simulink model "Suspension_system"  (R2023a)
settings: Solver=VariableStepAuto  StartTime=0.0  StopTime=10.0  RelTol=1e-3
values from neighbouring files (symbols this model uses):
  amp = 0.0025    [Parameters.m]
  c = 650    [Parameters.m]
  D_amp = 0.015    [Parameters.m]
  D_flat = 1    [Parameters.m]
  D_wave = 0.05    [Parameters.m]
  T_flat = 0.3048    [Parameters.m]    (also in task3.m; task4.m = 1)
  T_wave = 0.01    [Parameters.m]    (also in task3.m; task4.m = 0.05)
libraries: fl_lib x7, nesl_utility x4, simulink x1
settings Model: Creator=arnin  LastModifiedBy=arnin

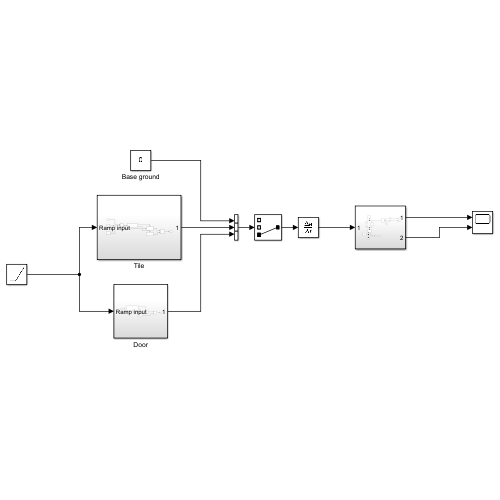
[thumbnail: Simulink's stored preview of the top-level diagram]
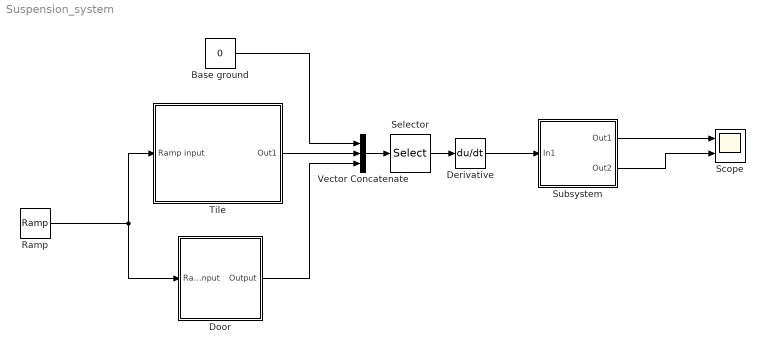
== system Suspension_system ==
  Base ground : Constant  Value=0
  Derivative : Derivative
  Door : Subsystem
  Ramp : simulink/Sources/Ramp  slope=3  start=0  InitialOutput=0
  Scope : Scope  NumInputPorts=2
  Selector : Selector  InputPortWidth=3  IndexOptions=Index vector (dialog)  Indices=[3]  OutputSizes=1
  Subsystem : Subsystem
  Tile : Subsystem
  Vector Concatenate : Concatenate  NumInputs=3
  wires:
  Ramp/1 -> Door/1(Ramp input), Tile/1(Ramp input)
  Base ground/1 -> Vector Concatenate/1
  Tile/1(Out1) -> Vector Concatenate/2
  Door/1(Output) -> Vector Concatenate/3
  Vector Concatenate/1 -> Selector/1
  Derivative/1 -> Subsystem/1(In1)
  Selector/1 -> Derivative/1
  Subsystem/1(Out1) -> Scope/1
  Subsystem/2(Out2) -> Scope/2

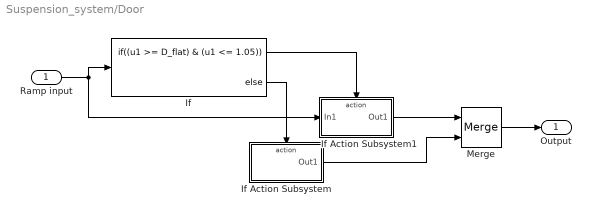
== system Suspension_system/Door ==
  Ramp input : Inport
  If : If  IfExpression=(u1 >= D_flat) & (u1 <= 1.05)
  If Action Subsystem : Subsystem  TreatAsAtomicUnit=on
  If Action Subsystem1 : Subsystem  TreatAsAtomicUnit=on
  Merge : Merge
  Output : Outport
  wires:
  If/2 -> If Action Subsystem/Action
  If Action Subsystem1/1(Out1) -> Merge/1
  Ramp input/1 -> If Action Subsystem1/1(In1), If/1
  If Action Subsystem/1(Out1) -> Merge/2
  If/1 -> If Action Subsystem1/Action
  Merge/1 -> Output/1

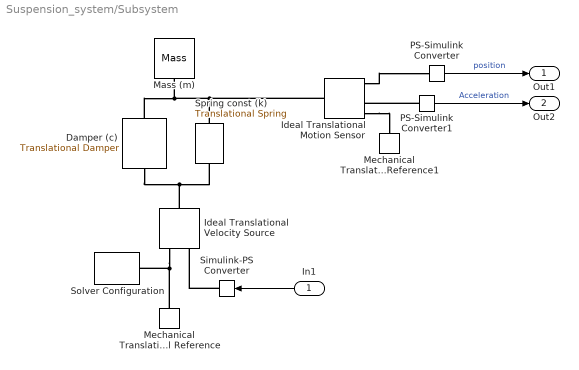
== system Suspension_system/Subsystem ==
  In1 : Inport
  Damper (c) : fl_lib/Mechanical/Translational Elements/Translational Damper  D=c N*s/m  v_specify=off  v_priority=None  v=0 m/s  v_nominal_specify=off  v_nominal_unit=m/s  v_nominal_value=1  f_specify=off  f_priority=None  f=0 N  f_nominal_specify=off  f_nominal_unit=N  f_nominal_value=1
  Ideal Translational Motion Sensor : fl_lib/Mechanical/Mechanical Sensors/Ideal Translational Motion Sensor  reference=foundation.enum.MeasurementReference.difference  acceleration_port=true  velocity_port=true  position_port=true  offset=0 m
      settings: InternalSimscapePortConfiguration="{\"Bottom\":[],\"Left\":[{\"id\":\"R\",\"label\":\"R\",\"type\":\"foundation.mechanical.translational.translational\"}],\"Right\":[{\"id\":\"C\",\"label\":\"C\",\"type\":\"foundation.mechanical.translational.translational\"},{\"id\":\"A\",\"label\":\"A\",\"type\":\"output\"},{\"id\":\"V\",\"label\":\"V\",\"type\":\"output\"},{\"id\":\"P\",\"label\":\"P\",\"type\":\"output\"}],\"Top\":[]}"
  Ideal Translational Velocity Source : fl_lib/Mechanical/Mechanical Sources/Ideal Translational Velocity Source
  Mass (m) : fl_lib/Mechanical/Translational Elements/Mass  mass=M kg  num_ports=foundation.enum.numPorts2.one  v_specify=off  v_priority=High  v=0 m/s  v_nominal_specify=off  v_nominal_unit=m/s  v_nominal_value=1  f_specify=off  f_priority=None  f=0 N  f_nominal_specify=off  f_nominal_unit=N  f_nominal_value=1
  Mechanical Translational Reference : fl_lib/Mechanical/Translational Elements/Mechanical Translational Reference
  Mechanical Translational Reference1 : fl_lib/Mechanical/Translational Elements/Mechanical Translational Reference
  PS-Simulink Converter : nesl_utility/PS-Simulink Converter  PhysicalDomain=network_engine_domain  SubClassName=ps_output  LeftPortType=input  RightPortType=output  PseudoPeriodic=off  Frequencies=[]  VectorFormat=inherit  Unit=inherit  AffineConversion=off
  PS-Simulink Converter1 : nesl_utility/PS-Simulink Converter  PhysicalDomain=network_engine_domain  SubClassName=ps_output  LeftPortType=input  RightPortType=output  PseudoPeriodic=off  Frequencies=[]  VectorFormat=inherit  Unit=inherit  AffineConversion=off
  Simulink-PS Converter : nesl_utility/Simulink-PS Converter  PhysicalDomain=network_engine_domain  SubClassName=ps_input  LeftPortType=input  RightPortType=output  PseudoPeriodic=off  Frequencies=[]  NoiseDistribution=none  NoiseParameters=[]  Unit=1  AffineConversion=off  FilteringAndDerivatives=provide  SimscapeFilterOrder=1  InputFilterTimeConstant=0.001  UdotUserProvided=0
  Solver Configuration : nesl_utility/Solver Configuration  PhysicalDomain=network_engine_domain  SubClassName=solver  LeftPortType=input  RightPortType=generic  Tones=[]  Harmonics=[]  SimulateNoise=off  Profile=off  UseLocalSampling=off  EnableSwitchedLinearOptims=on  FrequencyDomain=off  UseCCode=off  RelTol=0.001  AbsTol=0.001  MinStep=1e-09  ToWorkspace=off  RevertToSquareIcSolve=off  NumHomotopyIterations=100  PhasorMode=off  PhasorModeNumHarmonics=1  ConsistencySolver=NEWTON_XTOL_AFTER_FTOL  IndexReductionMethod=DerivativeReplacement  DoDC=off  ResidualTolerance=1e-09  ConsistencyTolSource=GLOBAL  ConsistencyAbsTol=0.001  ConsistencyRelTol=0.001  ConsistencyTolFactor=0.001  UseLocalSolver=off  LocalSolverChoice=NE_BACKWARD_EULER_ADVANCER  ResolveIndetEquations=on  FunctionEvalNumThread=1  LocalSolverSampleTime=0.001  DoFixedCost=off  MaxNonlinIter=3  MaxModeIter=2  ComputeImpulses=off  ImpulseIterations=2  LinearAlgebra=auto  LinearAlgebraNumThread=0  EquationFormulation=NE_TIME_EF  DelaysMemoryBudget=1024  AutomaticFiltering=on  FilteringTimeConstant=0.001  PartitionStorageMethod=AS_NEEDED  PartitionMemoryBudget=1024  PartitionMethod=ROBUST
  Spring const (k) : fl_lib/Mechanical/Translational Elements/Translational Spring  spr_rate=k N/m  v_specify=off  v_priority=None  v=0 m/s  v_nominal_specify=off  v_nominal_unit=m/s  v_nominal_value=1  f_specify=off  f_priority=None  f=0 N  f_nominal_specify=off  f_nominal_unit=N  f_nominal_value=1  x_specify=off  x_priority=High  x=0 m  x_nominal_specify=off  x_nominal_unit=m  x_nominal_value=1
  Out1 : Outport
  Out2 : Outport  Port=2
  wires:
  In1/1 -> Simulink-PS Converter/1
  PS-Simulink Converter1/1 -> Out2/1  "Acceleration"
  PS-Simulink Converter/1 -> Out1/1  "position"
  connections:
  Simulink-PS Converter/RConn1 -- Ideal Translational Velocity Source/RConn1
  Mechanical Translational Reference/LConn1 -- Solver Configuration/RConn1 -- Ideal Translational Velocity Source/RConn2
  Damper (c)/LConn1 -- Ideal Translational Motion Sensor/LConn1 -- Spring const (k)/LConn1 -- Mass (m)/LConn1
  Ideal Translational Motion Sensor/RConn4 -- PS-Simulink Converter/LConn1
  Damper (c)/RConn1 -- Ideal Translational Velocity Source/LConn1 -- Spring const (k)/RConn1
  Ideal Translational Motion Sensor/RConn1 -- Mechanical Translational Reference1/LConn1
  PS-Simulink Converter1/LConn1 -- Ideal Translational Motion Sensor/RConn2

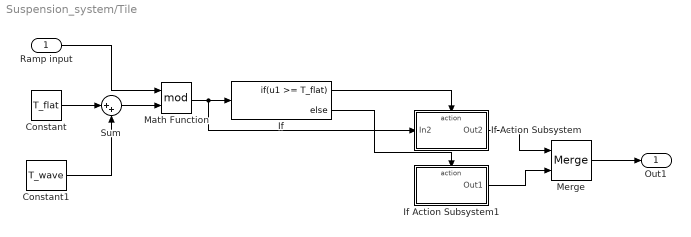
== system Suspension_system/Tile ==
  Ramp input : Inport
  Constant : Constant  Value=T_flat
  Constant1 : Constant  Value=T_wave
  If : If  IfExpression=u1 >= T_flat
  If Action Subsystem : Subsystem  TreatAsAtomicUnit=on
  If Action Subsystem1 : Subsystem  TreatAsAtomicUnit=on
  Math Function : Math  Operator=mod
  Merge : Merge
  Sum : Sum  Inputs=|++
  Out1 : Outport
  wires:
  Constant/1 -> Sum/1
  Constant1/1 -> Sum/2
  Sum/1 -> Math Function/2
  Ramp input/1 -> Math Function/1
  Math Function/1 -> If Action Subsystem/1(In2), If/1
  If/2 -> If Action Subsystem1/Action
  If Action Subsystem1/1(Out1) -> Merge/2
  If Action Subsystem/1(Out2) -> Merge/1
  Merge/1 -> Out1/1
  If/1 -> If Action Subsystem/Action

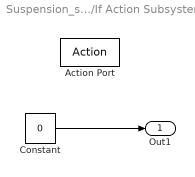
== system Suspension_system/Door/If Action Subsystem ==
  Action Port : ActionPort  ActionPortLabel=else
  Constant : Constant  Value=0
  Out1 : Outport
  wires:
  Constant/1 -> Out1/1

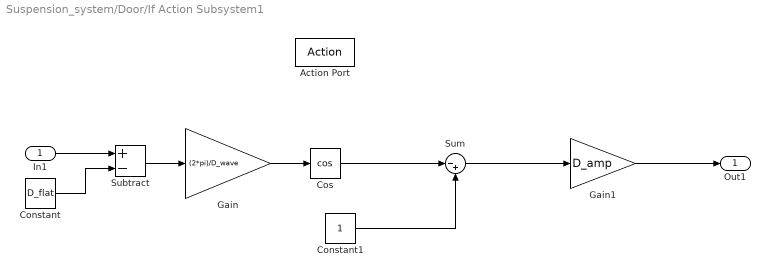
== system Suspension_system/Door/If Action Subsystem1 ==
  In1 : Inport
  Action Port : ActionPort  ActionPortLabel=if((u1 >= D_flat) & (u1 <= 1.05))
  Constant : Constant  Value=D_flat
  Constant1 : Constant
  Cos : Trigonometry  Operator=cos
  Gain : Gain  Gain=(2*pi)/D_wave
  Gain1 : Gain  Gain=D_amp
  Subtract : Sum  Inputs=+-
  Sum : Sum  Inputs=|-+
  Out1 : Outport
  wires:
  Sum/1 -> Gain1/1
  Gain1/1 -> Out1/1
  Cos/1 -> Sum/1
  Constant1/1 -> Sum/2
  Gain/1 -> Cos/1
  Constant/1 -> Subtract/2
  Subtract/1 -> Gain/1
  In1/1 -> Subtract/1

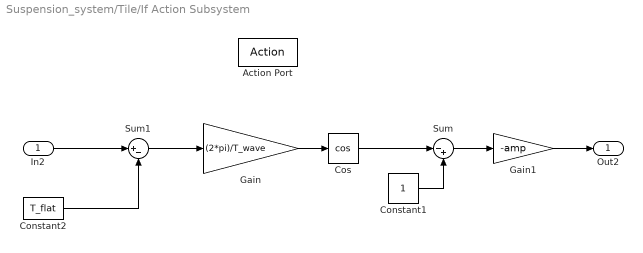
== system Suspension_system/Tile/If Action Subsystem ==
  In2 : Inport
  Action Port : ActionPort  ActionPortLabel=if(u1 >= T_flat)
  Constant1 : Constant
  Constant2 : Constant  Value=T_flat
  Cos : Trigonometry  Operator=cos
  Gain : Gain  Gain=(2*pi)/T_wave
  Gain1 : Gain  Gain=-amp
  Sum : Sum  Inputs=|-+
  Sum1 : Sum  Inputs=|+-
  Out2 : Outport
  wires:
  Sum/1 -> Gain1/1
  Cos/1 -> Sum/1
  Constant1/1 -> Sum/2
  In2/1 -> Sum1/1
  Gain/1 -> Cos/1
  Constant2/1 -> Sum1/2
  Sum1/1 -> Gain/1
  Gain1/1 -> Out2/1

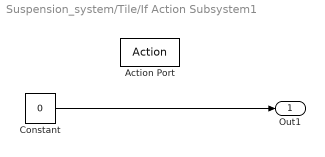
== system Suspension_system/Tile/If Action Subsystem1 ==
  Action Port : ActionPort  ActionPortLabel=else
  Constant : Constant  Value=0
  Out1 : Outport
  wires:
  Constant/1 -> Out1/1
